simulink model "baseline"  (R2025b)
settings: Solver=FixedStepDiscrete  StartTime=0  StopTime=0.72  FixedStep=0.08  RelTol=1e-3
InitFcn:
  | addpath(fileparts(get_param(bdroot,'FileName'))); init_baseline;
values from neighbouring files (symbols this model uses):
  cfg = evalin('base', 'cfg')    [baseline_step.m]    (also in init_baseline.m; run_baseline.m = init_baseline(); verify_baseline.m = init_baseline())
undefined symbols (not defined in the file or in its folder): baseline_step
settings Model: Creator=cherrywj  LastModifiedBy=cherrywj
settings DataIOCC: SaveOutput=off  SignalLogging=off

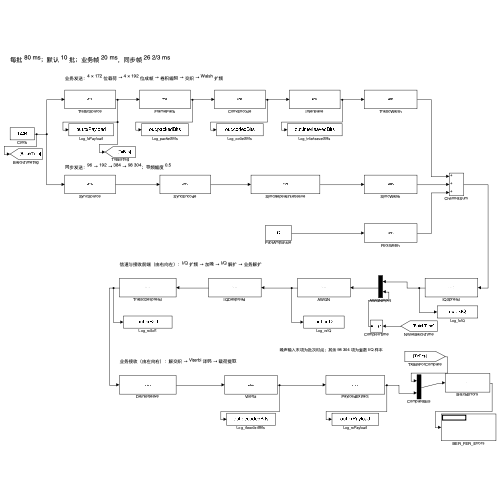
[thumbnail: Simulink's stored preview of the top-level diagram]
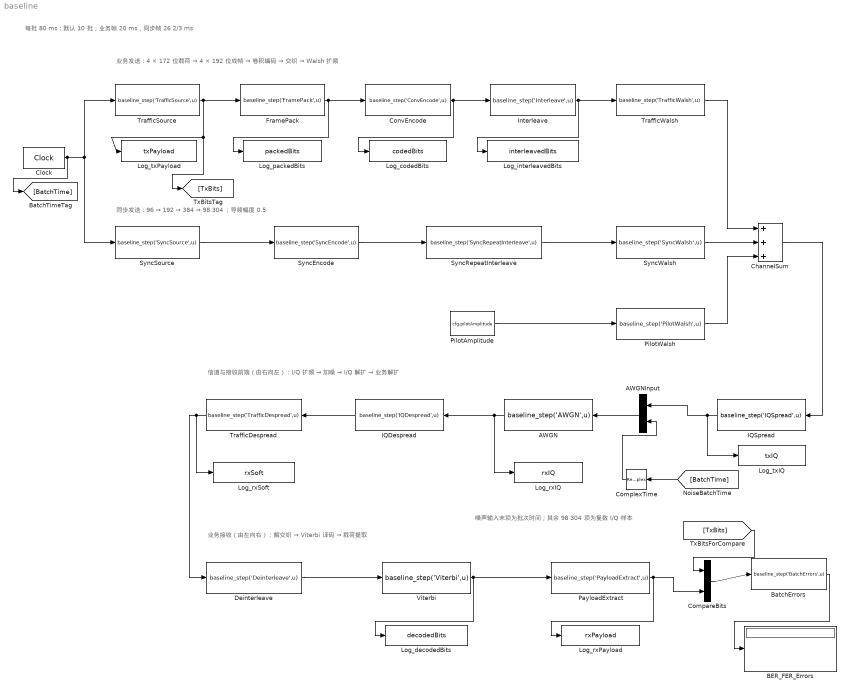
== system baseline ==
  note: 每批 80 ms；默认 10 批；业务帧 20 ms，同步帧 26 2/3 ms
  note: 业务发送：4 × 172 位载荷 → 4 × 192 位成帧 → 卷积编码 → 交织 → Walsh 扩频
  note: 同步发送：96 → 192 → 384 → 98 304；导频幅度 0.5
  note: 信道与接收前端（由右向左）：I/Q 扩频 → 加噪 → I/Q 解扩 → 业务解扩
  note: 噪声输入末项为批次时间；其余 98 304 项为复数 I/Q 样本
  note: 业务接收（由左向右）：解交织 → Viterbi 译码 → 载荷提取
  AWGN : MATLABFcn  MATLABFcn=baseline_step('AWGN',u)  OutputDimensions=98304  OutputSignalType=complex
  AWGNInput : Mux  Inputs=[98304 1]
  BER_FER_Errors : Display
  BatchErrors : MATLABFcn  MATLABFcn=baseline_step('BatchErrors',u)  OutputDimensions=3  OutputSignalType=real
  ChannelSum : Sum  Inputs=+++
  Clock : DigitalClock  SampleTime=0.08
  CompareBits : Mux  Inputs=[688 688]
  ComplexTime : RealImagToComplex  Input=Real
  ConvEncode : MATLABFcn  MATLABFcn=baseline_step('ConvEncode',u)  OutputDimensions=1536  OutputSignalType=real
  Deinterleave : MATLABFcn  MATLABFcn=baseline_step('Deinterleave',u)  OutputDimensions=1536  OutputSignalType=real
  FramePack : MATLABFcn  MATLABFcn=baseline_step('FramePack',u)  OutputDimensions=768  OutputSignalType=real
  IQDespread : MATLABFcn  MATLABFcn=baseline_step('IQDespread',u)  OutputDimensions=98304  OutputSignalType=real
  IQSpread : MATLABFcn  MATLABFcn=baseline_step('IQSpread',u)  OutputDimensions=98304  OutputSignalType=complex
  Interleave : MATLABFcn  MATLABFcn=baseline_step('Interleave',u)  OutputDimensions=1536  OutputSignalType=real
  Log_codedBits : ToWorkspace  VariableName=codedBits  SaveFormat=Timeseries  SampleTime=-1
  Log_decodedBits : ToWorkspace  VariableName=decodedBits  SaveFormat=Timeseries  SampleTime=-1
  Log_interleavedBits : ToWorkspace  VariableName=interleavedBits  SaveFormat=Timeseries  SampleTime=-1
  Log_packedBits : ToWorkspace  VariableName=packedBits  SaveFormat=Timeseries  SampleTime=-1
  Log_rxIQ : ToWorkspace  VariableName=rxIQ  SaveFormat=Timeseries  SampleTime=-1
  Log_rxPayload : ToWorkspace  VariableName=rxPayload  SaveFormat=Timeseries  SampleTime=-1
  Log_rxSoft : ToWorkspace  VariableName=rxSoft  SaveFormat=Timeseries  SampleTime=-1
  Log_txIQ : ToWorkspace  VariableName=txIQ  SaveFormat=Timeseries  SampleTime=-1
  Log_txPayload : ToWorkspace  VariableName=txPayload  SaveFormat=Timeseries  SampleTime=-1
  PayloadExtract : MATLABFcn  MATLABFcn=baseline_step('PayloadExtract',u)  OutputDimensions=688  OutputSignalType=real
  PilotAmplitude : Constant  Value=cfg.pilotAmplitude  OutDataTypeStr=double  SampleTime=0.08
  PilotWalsh : MATLABFcn  MATLABFcn=baseline_step('PilotWalsh',u)  OutputDimensions=98304  OutputSignalType=real
  SyncEncode : MATLABFcn  MATLABFcn=baseline_step('SyncEncode',u)  OutputDimensions=192  OutputSignalType=real
  SyncRepeatInterleave : MATLABFcn  MATLABFcn=baseline_step('SyncRepeatInterleave',u)  OutputDimensions=384  OutputSignalType=real
  SyncSource : MATLABFcn  MATLABFcn=baseline_step('SyncSource',u)  OutputDimensions=96  OutputSignalType=real
  SyncWalsh : MATLABFcn  MATLABFcn=baseline_step('SyncWalsh',u)  OutputDimensions=98304  OutputSignalType=real
  TrafficDespread : MATLABFcn  MATLABFcn=baseline_step('TrafficDespread',u)  OutputDimensions=1536  OutputSignalType=real
  TrafficSource : MATLABFcn  MATLABFcn=baseline_step('TrafficSource',u)  OutputDimensions=688  OutputSignalType=real
  TrafficWalsh : MATLABFcn  MATLABFcn=baseline_step('TrafficWalsh',u)  OutputDimensions=98304  OutputSignalType=real
  Viterbi : MATLABFcn  MATLABFcn=baseline_step('Viterbi',u)  OutputDimensions=768  OutputSignalType=real
  wires:
  Clock/1 -> TrafficSource/1, SyncSource/1, [BatchTime]
  TrafficSource/1 -> [TxBits], Log_txPayload/1, FramePack/1
  FramePack/1 -> ConvEncode/1, Log_packedBits/1
  ConvEncode/1 -> Interleave/1, Log_codedBits/1
  Interleave/1 -> TrafficWalsh/1, Log_interleavedBits/1
  SyncSource/1 -> SyncEncode/1
  SyncEncode/1 -> SyncRepeatInterleave/1
  SyncRepeatInterleave/1 -> SyncWalsh/1
  PilotAmplitude/1 -> PilotWalsh/1
  TrafficWalsh/1 -> ChannelSum/1
  SyncWalsh/1 -> ChannelSum/2
  PilotWalsh/1 -> ChannelSum/3
  ChannelSum/1 -> IQSpread/1
  IQSpread/1 -> AWGNInput/1, Log_txIQ/1
  [BatchTime] -> ComplexTime/1
  ComplexTime/1 -> AWGNInput/2
  AWGNInput/1 -> AWGN/1
  AWGN/1 -> IQDespread/1, Log_rxIQ/1
  IQDespread/1 -> TrafficDespread/1
  TrafficDespread/1 -> Deinterleave/1, Log_rxSoft/1
  Deinterleave/1 -> Viterbi/1
  Viterbi/1 -> PayloadExtract/1, Log_decodedBits/1
  [TxBits] -> CompareBits/1
  PayloadExtract/1 -> CompareBits/2, Log_rxPayload/1
  CompareBits/1 -> BatchErrors/1
  BatchErrors/1 -> BER_FER_Errors/1
